simulink model "Roll_Ap"  (R2012b)
settings: configuration reference "configSetObj_autopilot" (kept outside this file)
PostLoadFcn:
  | Roll_Ap_init
settings Model: RequirementInfo={} %GIDa_fe9045fd_0412_4b6e_8206_617cc20e6fde  CovSaveName=covdata_rollAP  CovMetricSettings=dcmtrwe  CovHTMLOptions=-aTS=1 -bRG=1 -bTC=1 -hTR=1 -nFC=0 -scm=1 -bcm=1  CovHtmlReporting=off  CovCumulativeVarName=covCumulativeData_rollAP  CovCumulativeReport=on  CovReportOnPause=off  CovModelRefEnable=on  Creator=bpotter  LastModifiedBy=ssauvage

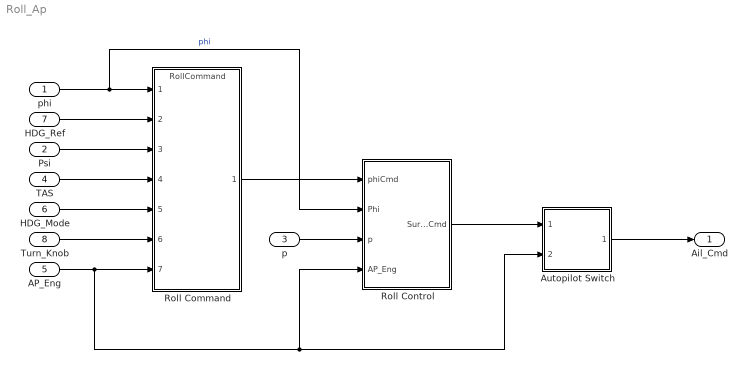
== system Roll_Ap ==
  phi : Inport  RequirementInfo={} %GIDa_040c2d73_6311_42f9_964f_56f1fff3d8d8  OutDataTypeStr=double  PortDimensions=1  SampleTime=1/40  Interpolate=off
  Psi : Inport  RequirementInfo={} %GIDa_aa699f91_96f0_401b_acdb_f9b4b0743533  Port=2  OutDataTypeStr=double  PortDimensions=1  SampleTime=1/40  Interpolate=off
  p : Inport  RequirementInfo={} %GIDa_91b6e343_cedd_4c09_9e82_9cc09e4312a7  Port=3  OutDataTypeStr=double  PortDimensions=1  SampleTime=1/40  Interpolate=off
  TAS : Inport  RequirementInfo={} %GIDa_9daa2c3d_09c1_4ac6_a206_1425f5f778cd  Port=4  OutDataTypeStr=double  PortDimensions=1  SampleTime=1/40  Interpolate=off
  AP_Eng : Inport  RequirementInfo={} %GIDa_dbf8c750_871c_42fc_8ea1_57838e97fa97  Port=5  OutDataTypeStr=boolean  PortDimensions=1  SampleTime=1/40  Interpolate=off
  HDG_Mode : Inport  RequirementInfo={} %GIDa_3d1fd2be_b046_42ef_8f3c_1955bceadbb7  Port=6  OutDataTypeStr=boolean  PortDimensions=1  SampleTime=1/40  Interpolate=off
  HDG_Ref : Inport  RequirementInfo={} %GIDa_96162cda_cb1a_490e_8dac_f861526aad50  Port=7  OutDataTypeStr=double  PortDimensions=1  SampleTime=1/40  Interpolate=off
  Turn_Knob : Inport  RequirementInfo={} %GIDa_fa976ccd_1ea9_4823_b673_fef2768ad601  Port=8  OutDataTypeStr=double  PortDimensions=1  SampleTime=1/40  Interpolate=off
  Autopilot Switch : Subsystem  RequirementInfo={} %GIDa_0338d8b4_919e_4053_80c0_5e0116df6a38
  Roll Command : ModelReference  ModelNameDialog=RollCommand  SimulationMode=Normal  ModelReferenceVersion=1.19  CopyOfModelName=RollCommand  DefaultDataLogging=on
  Roll Control : Subsystem
  Ail_Cmd : Outport  RequirementInfo={} %GIDa_02b61f6d_71d4_4b0d_89ac_bfbca808eb5f  OutDataTypeStr=double  PortDimensions=1  SampleTime=1/40
  wires:
  HDG_Ref/1 -> Roll Command/2
  phi/1 -> Roll Command/1, Roll Control/2(Phi)  "phi"
  p/1 -> Roll Control/3(p)
  Psi/1 -> Roll Command/3
  TAS/1 -> Roll Command/4
  Roll Command/1 -> Roll Control/1(phiCmd)
  HDG_Mode/1 -> Roll Command/5
  AP_Eng/1 -> Roll Command/7, Autopilot Switch/2(AP_Eng), Roll Control/4(AP_Eng)
  Roll Control/1(Surf_Cmd) -> Autopilot Switch/1(Surf_Cmd)
  Autopilot Switch/1(Ail_Cmd) -> Ail_Cmd/1
  Turn_Knob/1 -> Roll Command/6

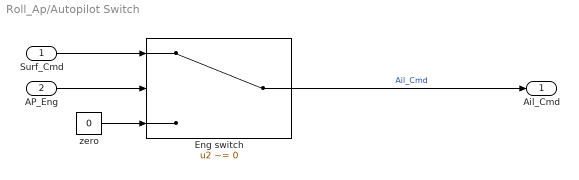
== system Roll_Ap/Autopilot Switch ==
  Surf_Cmd : Inport  OutDataTypeStr=double
  AP_Eng : Inport  Port=2  OutDataTypeStr=boolean
  Eng switch : Switch  RequirementInfo={} %GIDa_1f89e2a1_f10b_411b_80f1_4c7070559f04  Criteria=u2 ~= 0
      mask Display: disp('u2~=0')
  zero : Constant  RequirementInfo={} %GIDa_8c99e557_6257_4659_beae_770a67a6ac3a  Value=0  OutDataTypeStr=double
  Ail_Cmd : Outport
  wires:
  zero/1 -> Eng switch/3
  AP_Eng/1 -> Eng switch/2
  Surf_Cmd/1 -> Eng switch/1
  Eng switch/1 -> Ail_Cmd/1  "Ail_Cmd"

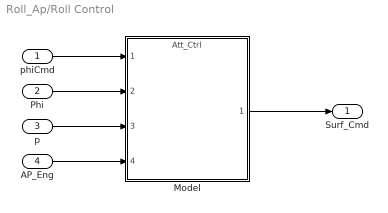
== system Roll_Ap/Roll Control ==
  phiCmd : Inport
  Phi : Inport  Port=2
  p : Inport  Port=3
  AP_Eng : Inport  Port=4
  Model : ModelReference  ModelNameDialog=Att_Ctrl  SimulationMode=Normal  ModelReferenceVersion=1.55  CopyOfModelName=Att_Ctrl  DefaultDataLogging=off
  Surf_Cmd : Outport
  wires:
  Phi/1 -> Model/2
  AP_Eng/1 -> Model/4
  phiCmd/1 -> Model/1
  Model/1 -> Surf_Cmd/1
  p/1 -> Model/3
